simulink model "Cv_03_2"  (R2022b)
settings: Solver=VariableStepAuto  StartTime=0.0  StopTime=10.0  RelTol=1e-3
model workspace (MAT data in the model file):
  t = 10
settings Model: Creator=honza  LastModifiedBy=honza
settings DataIOCC: ReturnWorkspaceOutputs=off

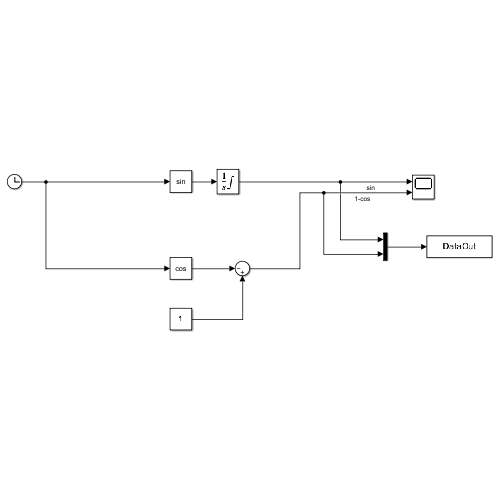
[thumbnail: Simulink's stored preview of the top-level diagram]
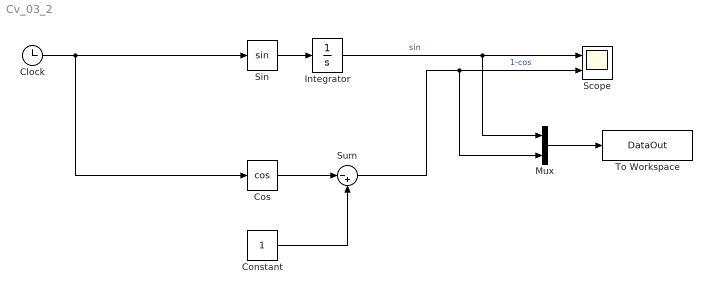
== system Cv_03_2 ==
  Clock : Clock
  Constant : Constant
  Cos : Trigonometry  Operator=cos
  Integrator : Integrator  LimitOutput=on  UpperSaturationLimit=10  LowerSaturationLimit=0
  Mux : Mux  Inputs=2
  Scope : Scope  NumInputPorts=2
  Sin : Trigonometry
  Sum : Sum  Inputs=|-+
  To Workspace : ToWorkspace  VariableName=DataOut  SampleTime=0.1
  wires:
  Clock/1 -> Sin/1, Cos/1
  Constant/1 -> Sum/2
  Cos/1 -> Sum/1
  Sum/1 -> Mux/2, Scope/2  "1-cos"
  Sin/1 -> Integrator/1
  Integrator/1 -> Mux/1, Scope/1  "sin"
  Mux/1 -> To Workspace/1
